simulink model "PlantControlR00"  (R2019a)
settings: Solver=VariableStepAuto  StartTime=0.0  StopTime=10.0  RelTol=1e-3
libraries: fl_lib x24, simulink x4, nesl_utility x2
settings Model: Creator=rjoseph  LastModifiedBy=rjoseph

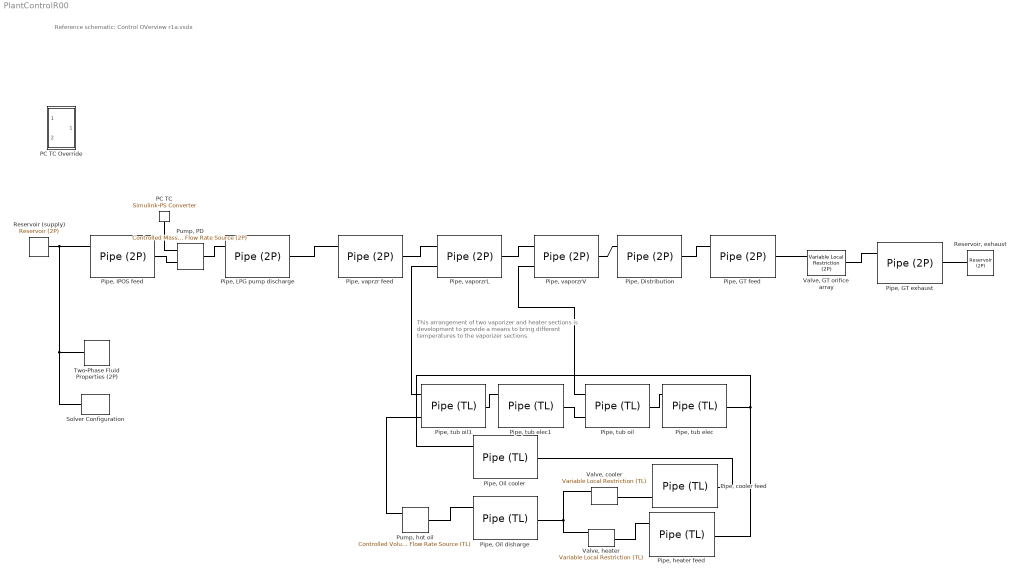
== system PlantControlR00 ==
  note: This arrangement of two vaporizer and heater sections
      | is development to provide a means to bring different
      | temperatures to the vaporizer sections.
  note: Reference schematic: Control OVerview r1a.vsdx
  PC TC : nesl_utility/Simulink-PS Converter  PhysicalDomain=network_engine_domain  SubClassName=ps_input  LeftPortType=input  RightPortType=output  PseudoPeriodic=off  Frequencies=[]  NoiseDistribution=none  NoiseParameters=[]  Unit=1  AffineConversion=off  FilteringAndDerivatives=provide  SimscapeFilterOrder=1  InputFilterTimeConstant=0.001  UdotUserProvided=0
  PC TC Override : Subsystem
  "Pipe, Distribution" : fl_lib/Two-Phase Fluid/Elements/Pipe (2P)  length=1300 ft  area=12.57 in^2  Dh=4 in  length_add=.5 ft  roughness=15e-4 in  Re_lam=2000  Re_tur=4000  shape_factor=64  Nu_lam=3.66  inertia=simscape.enum.onoff.off  energy_spec=foundation.enum.energy_spec.temperature  p_init=183 psi  T_init=85 degF  x_init=0  alpha_init=0.5  h_init=1500 kJ/kg  u_init=1500 kJ/kg  mdot_init=0 lbf/(ft/s)  time_constant=0.1 s
      settings: SourceProductName=Simscape  SourceProductBaseCode=SS
  "Pipe, GT exhaust" : fl_lib/Two-Phase Fluid/Elements/Pipe (2P)  length=1300 ft  area=12.57 in^2  Dh=4 in  length_add=.5 ft  roughness=15e-4 in  Re_lam=2000  Re_tur=4000  shape_factor=64  Nu_lam=3.66  inertia=simscape.enum.onoff.off  energy_spec=foundation.enum.energy_spec.temperature  p_init=183 psi  T_init=85 degF  x_init=0  alpha_init=0.5  h_init=1500 kJ/kg  u_init=1500 kJ/kg  mdot_init=0 lbf/(ft/s)  time_constant=0.1 s
      settings: SourceProductName=Simscape  SourceProductBaseCode=SS
  "Pipe, GT feed" : fl_lib/Two-Phase Fluid/Elements/Pipe (2P)  length=1300 ft  area=12.57 in^2  Dh=4 in  length_add=.5 ft  roughness=15e-4 in  Re_lam=2000  Re_tur=4000  shape_factor=64  Nu_lam=3.66  inertia=simscape.enum.onoff.off  energy_spec=foundation.enum.energy_spec.temperature  p_init=183 psi  T_init=85 degF  x_init=0  alpha_init=0.5  h_init=1500 kJ/kg  u_init=1500 kJ/kg  mdot_init=0 lbf/(ft/s)  time_constant=0.1 s
      settings: SourceProductName=Simscape  SourceProductBaseCode=SS
  "Pipe, IPOS feed" : fl_lib/Two-Phase Fluid/Elements/Pipe (2P)  length=1300 ft  area=12.57 in^2  Dh=4 in  length_add=.5 ft  roughness=15e-4 in  Re_lam=2000  Re_tur=4000  shape_factor=64  Nu_lam=3.66  inertia=simscape.enum.onoff.off  energy_spec=foundation.enum.energy_spec.temperature  p_init=183 psi  T_init=85 degF  x_init=0  alpha_init=0.5  h_init=1500 kJ/kg  u_init=1500 kJ/kg  mdot_init=0 lbf/(ft/s)  time_constant=0.1 s
      settings: SourceProductName=Simscape  SourceProductBaseCode=SS
  "Pipe, LPG pump discharge" : fl_lib/Two-Phase Fluid/Elements/Pipe (2P)  length=1300 ft  area=12.57 in^2  Dh=4 in  length_add=.5 ft  roughness=15e-4 in  Re_lam=2000  Re_tur=4000  shape_factor=64  Nu_lam=3.66  inertia=simscape.enum.onoff.off  energy_spec=foundation.enum.energy_spec.temperature  p_init=183 psi  T_init=85 degF  x_init=0  alpha_init=0.5  h_init=1500 kJ/kg  u_init=1500 kJ/kg  mdot_init=0 lbf/(ft/s)  time_constant=0.1 s
      settings: SourceProductName=Simscape  SourceProductBaseCode=SS
  "Pipe, Oil cooler" : fl_lib/Thermal Liquid/Elements/Pipe (TL)  dynamic_compressibility=simscape.enum.onoff.on  inertia=simscape.enum.onoff.off  length=5 m  area=0.01 m^2  Dh=0.1128 m  length_add=1 m  roughness=15e-6 m  Re_lam=2000  Re_tur=4000  shape_factor=64  Nu_lam=3.66  p0=0.101325 MPa  T0=293.15 K  mdot0=0 kg/s
      settings: SourceProductName=Simscape  SourceProductBaseCode=SS
  "Pipe, Oil disharge" : fl_lib/Thermal Liquid/Elements/Pipe (TL)  dynamic_compressibility=simscape.enum.onoff.on  inertia=simscape.enum.onoff.off  length=5 m  area=0.01 m^2  Dh=0.1128 m  length_add=1 m  roughness=15e-6 m  Re_lam=2000  Re_tur=4000  shape_factor=64  Nu_lam=3.66  p0=0.101325 MPa  T0=293.15 K  mdot0=0 kg/s
      settings: SourceProductName=Simscape  SourceProductBaseCode=SS
  "Pipe, cooler feed" : fl_lib/Thermal Liquid/Elements/Pipe (TL)  dynamic_compressibility=simscape.enum.onoff.on  inertia=simscape.enum.onoff.off  length=5 m  area=0.01 m^2  Dh=0.1128 m  length_add=1 m  roughness=15e-6 m  Re_lam=2000  Re_tur=4000  shape_factor=64  Nu_lam=3.66  p0=0.101325 MPa  T0=293.15 K  mdot0=0 kg/s
      settings: SourceProductName=Simscape  SourceProductBaseCode=SS
  "Pipe, heater feed" : fl_lib/Thermal Liquid/Elements/Pipe (TL)  dynamic_compressibility=simscape.enum.onoff.on  inertia=simscape.enum.onoff.off  length=5 m  area=0.01 m^2  Dh=0.1128 m  length_add=1 m  roughness=15e-6 m  Re_lam=2000  Re_tur=4000  shape_factor=64  Nu_lam=3.66  p0=0.101325 MPa  T0=293.15 K  mdot0=0 kg/s
      settings: SourceProductName=Simscape  SourceProductBaseCode=SS
  "Pipe, tub elec" : fl_lib/Thermal Liquid/Elements/Pipe (TL)  dynamic_compressibility=simscape.enum.onoff.on  inertia=simscape.enum.onoff.off  length=5 m  area=0.01 m^2  Dh=0.1128 m  length_add=1 m  roughness=15e-6 m  Re_lam=2000  Re_tur=4000  shape_factor=64  Nu_lam=3.66  p0=0.101325 MPa  T0=293.15 K  mdot0=0 kg/s
      settings: SourceProductName=Simscape  SourceProductBaseCode=SS
  "Pipe, tub elec1" : fl_lib/Thermal Liquid/Elements/Pipe (TL)  dynamic_compressibility=simscape.enum.onoff.on  inertia=simscape.enum.onoff.off  length=5 m  area=0.01 m^2  Dh=0.1128 m  length_add=1 m  roughness=15e-6 m  Re_lam=2000  Re_tur=4000  shape_factor=64  Nu_lam=3.66  p0=0.101325 MPa  T0=293.15 K  mdot0=0 kg/s
      settings: SourceProductName=Simscape  SourceProductBaseCode=SS
  "Pipe, tub oil" : fl_lib/Thermal Liquid/Elements/Pipe (TL)  dynamic_compressibility=simscape.enum.onoff.on  inertia=simscape.enum.onoff.off  length=5 m  area=0.01 m^2  Dh=0.1128 m  length_add=1 m  roughness=15e-6 m  Re_lam=2000  Re_tur=4000  shape_factor=64  Nu_lam=3.66  p0=0.101325 MPa  T0=293.15 K  mdot0=0 kg/s
      settings: SourceProductName=Simscape  SourceProductBaseCode=SS
  "Pipe, tub oil1" : fl_lib/Thermal Liquid/Elements/Pipe (TL)  dynamic_compressibility=simscape.enum.onoff.on  inertia=simscape.enum.onoff.off  length=5 m  area=0.01 m^2  Dh=0.1128 m  length_add=1 m  roughness=15e-6 m  Re_lam=2000  Re_tur=4000  shape_factor=64  Nu_lam=3.66  p0=0.101325 MPa  T0=293.15 K  mdot0=0 kg/s
      settings: SourceProductName=Simscape  SourceProductBaseCode=SS
  "Pipe, vaporzrL" : fl_lib/Two-Phase Fluid/Elements/Pipe (2P)  length=1300 ft  area=12.57 in^2  Dh=4 in  length_add=.5 ft  roughness=15e-4 in  Re_lam=2000  Re_tur=4000  shape_factor=64  Nu_lam=3.66  inertia=simscape.enum.onoff.off  energy_spec=foundation.enum.energy_spec.temperature  p_init=183 psi  T_init=85 degF  x_init=0  alpha_init=0.5  h_init=1500 kJ/kg  u_init=1500 kJ/kg  mdot_init=0 lbf/(ft/s)  time_constant=0.1 s
      settings: SourceProductName=Simscape  SourceProductBaseCode=SS
  "Pipe, vaporzrV" : fl_lib/Two-Phase Fluid/Elements/Pipe (2P)  length=1300 ft  area=12.57 in^2  Dh=4 in  length_add=.5 ft  roughness=15e-4 in  Re_lam=2000  Re_tur=4000  shape_factor=64  Nu_lam=3.66  inertia=simscape.enum.onoff.off  energy_spec=foundation.enum.energy_spec.temperature  p_init=183 psi  T_init=85 degF  x_init=0  alpha_init=0.5  h_init=1500 kJ/kg  u_init=1500 kJ/kg  mdot_init=0 lbf/(ft/s)  time_constant=0.1 s
      settings: SourceProductName=Simscape  SourceProductBaseCode=SS
  "Pipe, vaprzr feed" : fl_lib/Two-Phase Fluid/Elements/Pipe (2P)  length=1300 ft  area=12.57 in^2  Dh=4 in  length_add=.5 ft  roughness=15e-4 in  Re_lam=2000  Re_tur=4000  shape_factor=64  Nu_lam=3.66  inertia=simscape.enum.onoff.off  energy_spec=foundation.enum.energy_spec.temperature  p_init=183 psi  T_init=85 degF  x_init=0  alpha_init=0.5  h_init=1500 kJ/kg  u_init=1500 kJ/kg  mdot_init=0 lbf/(ft/s)  time_constant=0.1 s
      settings: SourceProductName=Simscape  SourceProductBaseCode=SS
  "Pump, PD" : fl_lib/Two-Phase Fluid/Sources/Controlled Mass Flow Rate Source (2P)  power_spec=foundation.enum.power_spec.isentropic  area_A=12.57 in^2  area_B=7.069 in^2
      settings: SourceProductName=Simscape  SourceProductBaseCode=SS
  "Pump, hot oil" : fl_lib/Thermal Liquid/Sources/Controlled Volumetric Flow Rate Source (TL)  area=0.01 m^2  length=0.1 m  mdot_A_specify=off  mdot_A_priority=None  mdot_A=1 kg/s  mdot_A_nominal_specify=off  mdot_A_nominal_unit=kg/s  mdot_A_nominal_value=1
      settings: SourceProductName=Simscape  SourceProductBaseCode=SS
  Reservoir (supply) : fl_lib/Two-Phase Fluid/Elements/Reservoir (2P)  pressure_spec=foundation.enum.pressure_spec.specified  reservoir_pressure=500 psi  energy_spec=foundation.enum.energy_spec.temperature  reservoir_temperature=85 degF  reservoir_quality=0.5  reservoir_void_fraction=0.5  reservoir_enthalpy=1500 kJ/kg  reservoir_internal_energy=1500 kJ/kg  area_A=2.96 in^2
      settings: SourceProductName=Simscape  SourceProductBaseCode=SS
  "Reservoir, exhaust" : fl_lib/Two-Phase Fluid/Elements/Reservoir (2P)  pressure_spec=foundation.enum.pressure_spec.specified  reservoir_pressure=550 psi  energy_spec=foundation.enum.energy_spec.temperature  reservoir_temperature=290 degF  reservoir_quality=0.5  reservoir_void_fraction=0.5  reservoir_enthalpy=1500 kJ/kg  reservoir_internal_energy=1500 kJ/kg  area_A=6.61 in^2
      settings: SourceProductName=Simscape  SourceProductBaseCode=SS
  Solver Configuration : nesl_utility/Solver Configuration  PhysicalDomain=network_engine_domain  SubClassName=solver  LeftPortType=input  RightPortType=generic  Tones=[]  Harmonics=[]  SimulateNoise=off  Profile=off  UseLocalSampling=off  EnableSwitchedLinearOptims=on  FrequencyDomain=off  UseCCode=off  RelTol=0.001  AbsTol=1e-06  MinStep=1e-09  ToWorkspace=off  RevertToSquareIcSolve=off  NumHomotopyIterations=100  PhasorMode=off  PhasorModeNumHarmonics=1  DoDC=off  ResidualTolerance=1e-02  UseLocalSolver=on  LocalSolverChoice=NE_BACKWARD_EULER_ADVANCER  LocalSolverSampleTime=.005  DoFixedCost=off  MaxNonlinIter=3  MaxModeIter=2  LinearAlgebra=auto  EquationFormulation=NE_TIME_EF  DelaysMemoryBudget=1024  AutomaticFiltering=off  FilteringTimeConstant=0.001  PartitionStorageMethod=AS_NEEDED  PartitionMemoryBudget=1024  PartitionMethod=FAST
  Two-Phase Fluid Properties (2P) : fl_lib/Two-Phase Fluid/Utilities/Two-Phase Fluid Properties (2P)  u_min=C3H8Tables.u_min kJ/kg  u_max=C3H8Tables.u_max kJ/kg  unorm_liq=C3H8Tables.liquid.unorm  unorm_vap=C3H8Tables.vapor.unorm  p_TLU=C3H8Tables.p MPa  v_liq=C3H8Tables.liquid.v m^3/kg  v_vap=C3H8Tables.vapor.v m^3/kg  s_liq=C3H8Tables.liquid.s kJ/(kg*K)  s_vap=C3H8Tables.vapor.s kJ/(kg*K)  T_liq=C3H8Tables.liquid.T K  T_vap=C3H8Tables.vapor.T K  nu_liq=C3H8Tables.liquid.nu mm^2/s  nu_vap=C3H8Tables.vapor.nu mm^2/s  k_liq=C3H8Tables.liquid.k W/(m*K)  k_vap=C3H8Tables.vapor.k W/(m*K)  Pr_liq=C3H8Tables.liquid.Pr  Pr_vap=C3H8Tables.vapor.Pr  u_sat_liq=C3H8Tables.liquid.u_sat kJ/kg  u_sat_vap=C3H8Tables.vapor.u_sat kJ/kg  p_crit=C3H8Tables.p_crit MPa  critical_region=foundation.enum.critical_region.clip  p_crit_fraction=0.12  p_atm=0.101325 MPa  q_rev=0.01 Pa
      settings: SourceProductName=Simscape  SourceProductBaseCode=SS
  "Valve, GT orifice array" : fl_lib/Two-Phase Fluid/Elements/Variable Local Restriction (2P)  min_area=1e-10 m^2  max_area=0.005 m^2  area=0.01 m^2  Cd=0.64  B_lam=0.999
      settings: SourceProductName=Simscape  SourceProductBaseCode=SS
  "Valve, cooler" : fl_lib/Thermal Liquid/Elements/Variable Local Restriction (TL)  min_area=1e-10 m^2  max_area=0.005 m^2  area=0.01 m^2  length=0.1 m  Cd=0.7  pressure_recovery=1  Re_c=12  mdot_A_specify=off  mdot_A_priority=None  mdot_A=1 kg/s  mdot_A_nominal_specify=off  mdot_A_nominal_unit=kg/s  mdot_A_nominal_value=1
      settings: SourceProductName=Simscape  SourceProductBaseCode=SS
  "Valve, heater" : fl_lib/Thermal Liquid/Elements/Variable Local Restriction (TL)  min_area=1e-10 m^2  max_area=0.005 m^2  area=0.01 m^2  length=0.1 m  Cd=0.7  pressure_recovery=1  Re_c=12  mdot_A_specify=off  mdot_A_priority=None  mdot_A=1 kg/s  mdot_A_nominal_specify=off  mdot_A_nominal_unit=kg/s  mdot_A_nominal_value=1
      settings: SourceProductName=Simscape  SourceProductBaseCode=SS
  wires:
  ? -> PC TC/1
  connections:
  "Pump, PD"/RConn1 -- "Pipe, LPG pump discharge"/LConn1
  "Pipe, IPOS feed"/RConn1 -- "Pump, PD"/LConn1
  "Pipe, vaprzr feed"/LConn1 -- "Pipe, LPG pump discharge"/RConn1
  "Pipe, vaprzr feed"/RConn1 -- "Pipe, vaporzrL"/LConn1
  "Pipe, Distribution"/RConn1 -- "Pipe, GT feed"/LConn1
  "Pipe, tub oil1"/LConn1 -- "Pump, hot oil"/LConn1
  "Pump, hot oil"/RConn1 -- "Pipe, Oil disharge"/LConn1
  "Pipe, Oil disharge"/RConn1 -- "Valve, cooler"/LConn1 -- "Valve, heater"/LConn1
  "Pipe, cooler feed"/RConn1 -- "Pipe, Oil cooler"/RConn1
  "Pipe, heater feed"/RConn1 -- "Pipe, Oil cooler"/LConn1 -- "Pipe, tub elec"/RConn1
  "Valve, cooler"/RConn1 -- "Pipe, cooler feed"/LConn1
  "Valve, heater"/RConn1 -- "Pipe, heater feed"/LConn1
  "Pipe, vaporzrL"/RConn1 -- "Pipe, vaporzrV"/LConn1
  "Pipe, vaporzrV"/RConn1 -- "Pipe, Distribution"/LConn1
  "Pipe, tub oil"/RConn1 -- "Pipe, tub elec"/LConn1
  "Pipe, tub oil"/LConn1 -- "Pipe, tub elec1"/RConn1
  "Pipe, tub elec1"/LConn1 -- "Pipe, tub oil1"/RConn1
  "Pipe, tub oil"/LConn2 -- "Pipe, vaporzrV"/LConn2
  "Pipe, tub oil1"/LConn2 -- "Pipe, vaporzrL"/LConn2
  "Pipe, GT feed"/RConn1 -- "Valve, GT orifice array"/LConn1
  "Pipe, GT exhaust"/LConn1 -- "Valve, GT orifice array"/RConn1
  Solver Configuration/RConn1 -- Two-Phase Fluid Properties (2P)/RConn1 -- Reservoir (supply)/LConn1 -- "Pipe, IPOS feed"/LConn1
  "Pipe, GT exhaust"/RConn1 -- "Reservoir, exhaust"/LConn1
  PC TC/RConn1 -- "Pump, PD"/LConn2

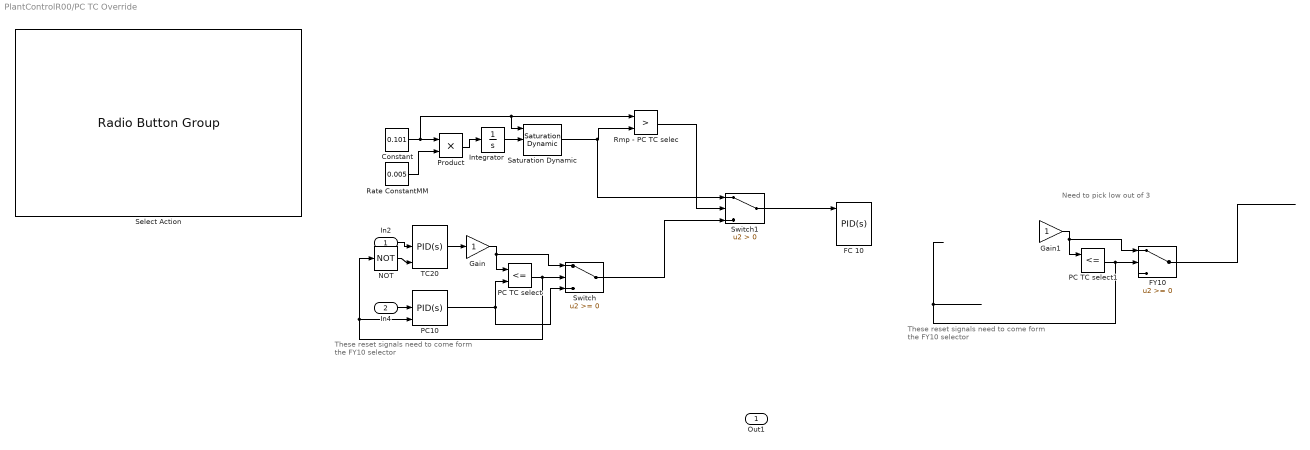
== system PlantControlR00/PC TC Override ==
  note: Need to pick low out of 3
  note: These reset signals need to come form
      | the FY10 selector
  note: These reset signals need to come form
      | the FY10 selector
  In2 : Inport
  In4 : Inport  Port=2
  Constant : Constant  Value=0.101
  FC 10 : simulink/Continuous/PID Controller (2DOF)  Controller=PID  Form=Parallel  TimeDomain=Continuous-time  SampleTime=-1  IntegratorMethod=Forward Euler  FilterMethod=Forward Euler  ControllerParametersSource=internal  P=1  I=1  D=0  UseFilter=on  N=100  b=1  c=1  TunerSelectOption=Transfer Function Based (PID Tuner App)  InitialConditionSource=internal  InitialConditionForIntegrator=0  InitialConditionForFilter=0  DifferentiatorICPrevScaledInput=0  ExternalReset=none  TrackingMode=on  Kt=1  LimitOutput=on  UpperSaturationLimit=10  LowerSaturationLimit=10  LinearizeAsGain=on  AntiWindupMode=clamping  Kb=1  POutMin=[]  POutMax=[]  IOutMin=[]  IOutMax=[]  DOutMin=[]  DOutMax=[]  NOutMin=[]  NOutMax=[]  bOutMin=[]  bOutMax=[]  cOutMin=[]  cOutMax=[]  SumOutMin=[]  SumOutMax=[]  SaturationOutMin=[]  SaturationOutMax=[]  PParamMin=[]  PParamMax=[]  IParamMin=[]  IParamMax=[]  DParamMin=[]  DParamMax=[]  NParamMin=[]  NParamMax=[]  bParamMin=[]  bParamMax=[]  cParamMin=[]  cParamMax=[]  KbParamMin=[]  KbParamMax=[]  KtParamMin=[]  KtParamMax=[]  KbOutMin=[]  KbOutMax=[]  KtOutMin=[]  KtOutMax=[]  IntegratorOutMin=[]  IntegratorOutMax=[]  FilterOutMin=[]  FilterOutMax=[]  SumI1OutMin=[]  SumI1OutMax=[]  SumI2OutMin=[]  SumI2OutMax=[]  SumI3OutMin=[]  SumI3OutMax=[]  SumI4OutMin=[]  SumI4OutMax=[]  SumDOutMin=[]  SumDOutMax=[]  Sum1OutMin=[]  Sum1OutMax=[]  Sum2OutMin=[]  Sum2OutMax=[]  Sum3OutMin=[]  Sum3OutMax=[]  DifferentiatorOutMin=[]  DifferentiatorOutMax=[]  FilterDiffOutCoefMin=[]  FilterDiffOutCoefMax=[]  ReciprocalOutMin=[]  ReciprocalOutMax=[]  SumDenOutMin=[]  SumDenOutMax=[]  SumNumOutMin=[]  SumNumOutMax=[]  DivideOutMin=[]  DivideOutMax=[]  IntegratorContinuousStateAttributes=''  IntegratorStateMustResolveToSignalObject=off  IntegratorRTWStateStorageClass=Auto  FilterContinuousStateAttributes=''  FilterStateMustResolveToSignalObject=off  FilterRTWStateStorageClass=Auto  ParallelPVariant=InternalParameters  IdealPVariant=Disabled  IVariant=InternalParameters  DVariant=InternalParameters  bVariant=InternalParameters  cVariant=InternalParameters  IntegratorVariant=Continuous  SatVariant=Enabled  AWVariant=ContClampingParallel  PCopyVariant=Disabled  TRVariant=Enabled  FdbkBlocksVariant=Forward  IdealPFdbkVariant=Disabled  SatFdbkVariant=Disabled  DerivativeFilterVariant=ContFilter  NVariant=InternalParameters  NCopyVariant=Disabled  FilterICVariant=InternalICsFilter  IntegratorICVariant=InternalICs  ExternalResetVariant=Disabled  TRSumVariant=TrackingMode  SumFdbkVariant=Disabled  SumVariant=Sum_PID
  FY10 : Switch
  Gain : Gain
  Gain1 : Gain
  Integrator : Integrator  ZeroCross=off
  NOT : Logic  Operator=NOT  IconShape=distinctive  AllPortsSameDT=off  OutDataTypeStr=boolean
  PC TC select : RelationalOperator  Operator=<=  OutDataTypeStr=boolean  RndMeth=Simplest
  PC TC select1 : RelationalOperator  Operator=<=  OutDataTypeStr=boolean  RndMeth=Simplest
  PC10 : simulink/Continuous/PID Controller (2DOF)  Controller=PID  Form=Parallel  TimeDomain=Continuous-time  SampleTime=-1  IntegratorMethod=Forward Euler  FilterMethod=Forward Euler  ControllerParametersSource=internal  P=1  I=1  D=0  UseFilter=on  N=100  b=1  c=1  TunerSelectOption=Transfer Function Based (PID Tuner App)  InitialConditionSource=internal  InitialConditionForIntegrator=0  InitialConditionForFilter=0  DifferentiatorICPrevScaledInput=0  ExternalReset=none  TrackingMode=on  Kt=1  LimitOutput=on  UpperSaturationLimit=10  LowerSaturationLimit=10  LinearizeAsGain=on  AntiWindupMode=clamping  Kb=1  POutMin=[]  POutMax=[]  IOutMin=[]  IOutMax=[]  DOutMin=[]  DOutMax=[]  NOutMin=[]  NOutMax=[]  bOutMin=[]  bOutMax=[]  cOutMin=[]  cOutMax=[]  SumOutMin=[]  SumOutMax=[]  SaturationOutMin=[]  SaturationOutMax=[]  PParamMin=[]  PParamMax=[]  IParamMin=[]  IParamMax=[]  DParamMin=[]  DParamMax=[]  NParamMin=[]  NParamMax=[]  bParamMin=[]  bParamMax=[]  cParamMin=[]  cParamMax=[]  KbParamMin=[]  KbParamMax=[]  KtParamMin=[]  KtParamMax=[]  KbOutMin=[]  KbOutMax=[]  KtOutMin=[]  KtOutMax=[]  IntegratorOutMin=[]  IntegratorOutMax=[]  FilterOutMin=[]  FilterOutMax=[]  SumI1OutMin=[]  SumI1OutMax=[]  SumI2OutMin=[]  SumI2OutMax=[]  SumI3OutMin=[]  SumI3OutMax=[]  SumI4OutMin=[]  SumI4OutMax=[]  SumDOutMin=[]  SumDOutMax=[]  Sum1OutMin=[]  Sum1OutMax=[]  Sum2OutMin=[]  Sum2OutMax=[]  Sum3OutMin=[]  Sum3OutMax=[]  DifferentiatorOutMin=[]  DifferentiatorOutMax=[]  FilterDiffOutCoefMin=[]  FilterDiffOutCoefMax=[]  ReciprocalOutMin=[]  ReciprocalOutMax=[]  SumDenOutMin=[]  SumDenOutMax=[]  SumNumOutMin=[]  SumNumOutMax=[]  DivideOutMin=[]  DivideOutMax=[]  IntegratorContinuousStateAttributes=''  IntegratorStateMustResolveToSignalObject=off  IntegratorRTWStateStorageClass=Auto  FilterContinuousStateAttributes=''  FilterStateMustResolveToSignalObject=off  FilterRTWStateStorageClass=Auto  ParallelPVariant=InternalParameters  IdealPVariant=Disabled  IVariant=InternalParameters  DVariant=InternalParameters  bVariant=InternalParameters  cVariant=InternalParameters  IntegratorVariant=Continuous  SatVariant=Enabled  AWVariant=ContClampingParallel  PCopyVariant=Disabled  TRVariant=Enabled  FdbkBlocksVariant=Forward  IdealPFdbkVariant=Disabled  SatFdbkVariant=Disabled  DerivativeFilterVariant=ContFilter  NVariant=InternalParameters  NCopyVariant=Disabled  FilterICVariant=InternalICsFilter  IntegratorICVariant=InternalICs  ExternalResetVariant=Disabled  TRSumVariant=TrackingMode  SumFdbkVariant=Disabled  SumVariant=Sum_PID
  Product : Product
  Rate ConstantMM : Constant  Value=0.005
  Rmp - PC TC selec : RelationalOperator  Operator=>  OutDataTypeStr=boolean  RndMeth=Simplest
  Saturation Dynamic : simulink/Discontinuities/Saturation Dynamic  OutMin=0  OutMax=[]  OutDataTypeStr=Inherit: Same as second input  OutDataType=fixdt(1, 16)  OutScaling=2^-10  DoSatur=off
  Select Action : RadioButtonGroup  SelectedLabel=Ramp to Start  ButtonGroupName=Flow Rate
      settings: Values={{'Ramp to Start', 'Ramp to Idle'}, [0.101 0.202]}
  Switch : Switch
  Switch1 : Switch  Criteria=u2 > Threshold
  TC20 : simulink/Continuous/PID Controller (2DOF)  Controller=PID  Form=Parallel  TimeDomain=Continuous-time  SampleTime=-1  IntegratorMethod=Forward Euler  FilterMethod=Forward Euler  ControllerParametersSource=internal  P=1  I=1  D=0  UseFilter=on  N=100  b=1  c=1  TunerSelectOption=Transfer Function Based (PID Tuner App)  InitialConditionSource=internal  InitialConditionForIntegrator=0  InitialConditionForFilter=0  DifferentiatorICPrevScaledInput=0  ExternalReset=none  TrackingMode=on  Kt=1  LimitOutput=on  UpperSaturationLimit=10  LowerSaturationLimit=10  LinearizeAsGain=on  AntiWindupMode=clamping  Kb=1  POutMin=[]  POutMax=[]  IOutMin=[]  IOutMax=[]  DOutMin=[]  DOutMax=[]  NOutMin=[]  NOutMax=[]  bOutMin=[]  bOutMax=[]  cOutMin=[]  cOutMax=[]  SumOutMin=[]  SumOutMax=[]  SaturationOutMin=[]  SaturationOutMax=[]  PParamMin=[]  PParamMax=[]  IParamMin=[]  IParamMax=[]  DParamMin=[]  DParamMax=[]  NParamMin=[]  NParamMax=[]  bParamMin=[]  bParamMax=[]  cParamMin=[]  cParamMax=[]  KbParamMin=[]  KbParamMax=[]  KtParamMin=[]  KtParamMax=[]  KbOutMin=[]  KbOutMax=[]  KtOutMin=[]  KtOutMax=[]  IntegratorOutMin=[]  IntegratorOutMax=[]  FilterOutMin=[]  FilterOutMax=[]  SumI1OutMin=[]  SumI1OutMax=[]  SumI2OutMin=[]  SumI2OutMax=[]  SumI3OutMin=[]  SumI3OutMax=[]  SumI4OutMin=[]  SumI4OutMax=[]  SumDOutMin=[]  SumDOutMax=[]  Sum1OutMin=[]  Sum1OutMax=[]  Sum2OutMin=[]  Sum2OutMax=[]  Sum3OutMin=[]  Sum3OutMax=[]  DifferentiatorOutMin=[]  DifferentiatorOutMax=[]  FilterDiffOutCoefMin=[]  FilterDiffOutCoefMax=[]  ReciprocalOutMin=[]  ReciprocalOutMax=[]  SumDenOutMin=[]  SumDenOutMax=[]  SumNumOutMin=[]  SumNumOutMax=[]  DivideOutMin=[]  DivideOutMax=[]  IntegratorContinuousStateAttributes=''  IntegratorStateMustResolveToSignalObject=off  IntegratorRTWStateStorageClass=Auto  FilterContinuousStateAttributes=''  FilterStateMustResolveToSignalObject=off  FilterRTWStateStorageClass=Auto  ParallelPVariant=InternalParameters  IdealPVariant=Disabled  IVariant=InternalParameters  DVariant=InternalParameters  bVariant=InternalParameters  cVariant=InternalParameters  IntegratorVariant=Continuous  SatVariant=Enabled  AWVariant=ContClampingParallel  PCopyVariant=Disabled  TRVariant=Enabled  FdbkBlocksVariant=Forward  IdealPFdbkVariant=Disabled  SatFdbkVariant=Disabled  DerivativeFilterVariant=ContFilter  NVariant=InternalParameters  NCopyVariant=Disabled  FilterICVariant=InternalICsFilter  IntegratorICVariant=InternalICs  ExternalResetVariant=Disabled  TRSumVariant=TrackingMode  SumFdbkVariant=Disabled  SumVariant=Sum_PID
  Out1 : Outport
  wires:
  PC TC select/1 -> Switch/2, PC10/3, NOT/1
  PC10/1 -> PC TC select/2, Switch/3
  Gain/1 -> PC TC select/1, Switch/1
  TC20/1 -> Gain/1
  In2/1 -> TC20/2
  NOT/1 -> TC20/3
  Switch/1 -> Switch1/3
  In4/1 -> PC10/2
  Product/1 -> Integrator/1
  Integrator/1 -> Saturation Dynamic/2
  Rate ConstantMM/1 -> Product/2
  Constant/1 -> Product/1, Rmp - PC TC selec/1, Saturation Dynamic/1
  Saturation Dynamic/1 -> Switch1/1, Rmp - PC TC selec/2
  Rmp - PC TC selec/1 -> Switch1/2
  Switch1/1 -> FC 10/1
  FY10/1 -> ?
  Gain1/1 -> PC TC select1/1, FY10/1
  ? -> Gain1/1
  PC TC select1/1 -> FY10/2
  ? -> PC TC select1/2, FY10/3
